simulink model "TALLER5"  (R2023b)
settings: Solver=VariableStepAuto  StartTime=0.0  StopTime=0.25  RelTol=1e-3
undefined symbols (not defined in the file): Cap, den, Kd3, Ki3, Kp2, Kp3, L, num, R
libraries: simulink x9, slpidlib x1
settings Model: Creator=Gabbi C  LastModifiedBy=Gabbi C

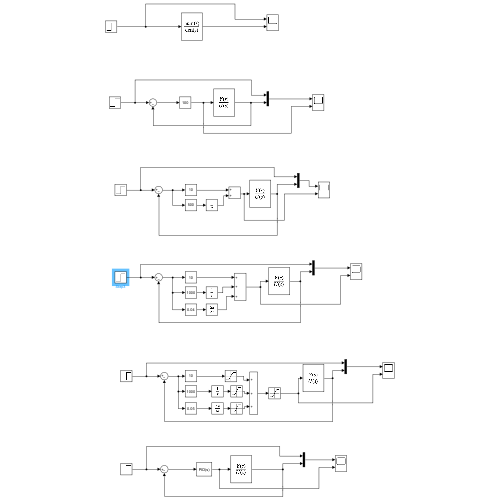
[thumbnail: Simulink's stored preview of the top-level diagram]
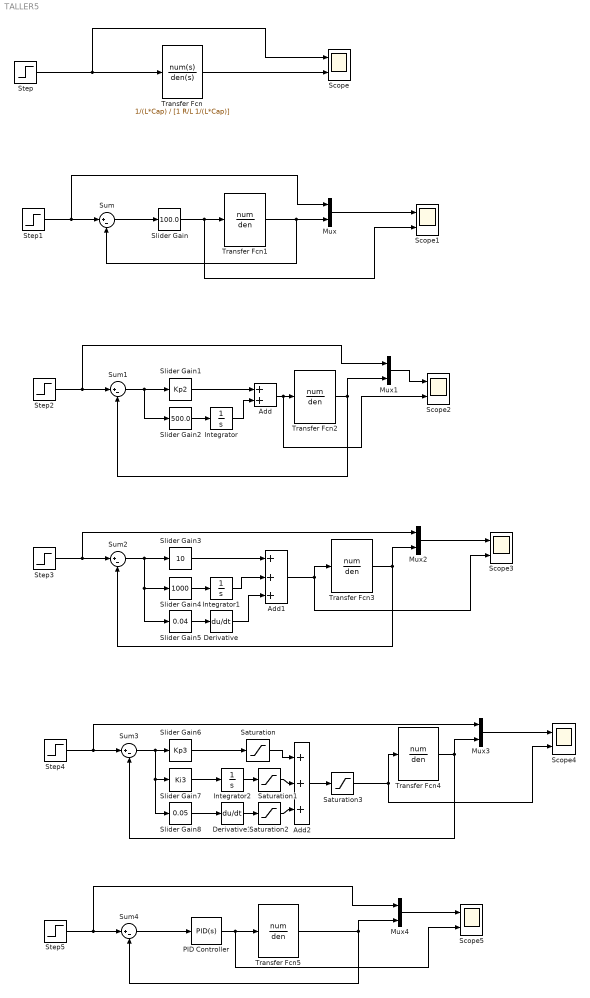
== system TALLER5 ==
  Add : Sum
  Add1 : Sum  Inputs=+++
  Add2 : Sum  Inputs=+++
  Derivative : Derivative
  Derivative1 : Derivative
  Integrator : Integrator
  Integrator1 : Integrator
  Integrator2 : Integrator
  Mux{,1..4} (5 alike) : Mux  Inputs=2
  PID Controller : slpidlib/PID Controller  Controller=PID  Form=Parallel  TimeDomain=Continuous-time  UseExternalTs=off  SampleTime=-1  IntegratorMethod=Forward Euler  FilterMethod=Forward Euler  ControllerParametersSource=internal  P=Kp3  I=Ki3  UseKiTs=off  D=Kd3  N=1000000  UseFilter=on  TunerSelectOption=Transfer Function Based (PID Tuner App)  InitialConditionSource=internal  InitialConditionForIntegrator=0  InitialConditionForFilter=0  DifferentiatorICPrevScaledInput=0  ExternalReset=none  TrackingMode=off  Kt=1  LimitOutput=off  SatLimitsSource=internal  UpperSaturationLimit=inf  LowerSaturationLimit=-inf  LinearizeAsGain=on  AntiWindupMode=none  Kb=1  LimitIntegrator=off  UpperIntegratorSaturationLimit=inf  LowerIntegratorSaturationLimit=-inf  POutMin=[]  POutMax=[]  IOutMin=[]  IOutMax=[]  DOutMin=[]  DOutMax=[]  NOutMin=[]  NOutMax=[]  SumOutMin=[]  SumOutMax=[]  SaturationOutMin=[]  SaturationOutMax=[]  PParamMin=[]  PParamMax=[]  IParamMin=[]  IParamMax=[]  DParamMin=[]  DParamMax=[]  NParamMin=[]  NParamMax=[]  KbParamMin=[]  KbParamMax=[]  KtParamMin=[]  KtParamMax=[]  KbOutMin=[]  KbOutMax=[]  KtOutMin=[]  KtOutMax=[]  IntegratorOutMin=[]  IntegratorOutMax=[]  FilterOutMin=[]  FilterOutMax=[]  SumI1OutMin=[]  SumI1OutMax=[]  SumI2OutMin=[]  SumI2OutMax=[]  SumI3OutMin=[]  SumI3OutMax=[]  SumI4OutMin=[]  SumI4OutMax=[]  SumDOutMin=[]  SumDOutMax=[]  DifferentiatorOutMin=[]  DifferentiatorOutMax=[]  FilterDiffOutCoefMin=[]  FilterDiffOutCoefMax=[]  ReciprocalOutMin=[]  ReciprocalOutMax=[]  SumDenOutMin=[]  SumDenOutMax=[]  SumNumOutMin=[]  SumNumOutMax=[]  DivideOutMin=[]  DivideOutMax=[]  UdiffTsProdOutMin=[]  UdiffTsProdOutMax=[]  NTsProdOutMin=[]  NTsProdOutMax=[]  UintegralTsProdOutMin=[]  UintegralTsProdOutMax=[]  UngainTsProdOutMin=[]  UngainTsProdOutMax=[]  ClampingZeroOutDataTypeStr=Inherit: Inherit via back propagation  ClampingZeroOutMin=[]  ClampingZeroOutMax=[]  FilterDenConstantOutDataTypeStr=Inherit: Inherit via back propagation  FilterDenConstantOutMin=[]  FilterDenConstantOutMax=[]  PCopyOutDataTypeStr=Inherit: Inherit via back propagation  PCopyOutMin=[]  PCopyOutMax=[]  NCopyOutDataTypeStr=Inherit: Inherit via back propagation  NCopyOutMin=[]  NCopyOutMax=[]  IntegratorContinuousStateAttributes=''  IntegratorStateMustResolveToSignalObject=off  IntegratorRTWStateStorageClass=Auto  FilterContinuousStateAttributes=''  FilterStateMustResolveToSignalObject=off  FilterRTWStateStorageClass=Auto  ParallelPVariant=InternalParameters  IdealPVariant=Disabled  IVariant=InternalParameters  DVariant=InternalParameters  IntegratorVariant=Continuous  SatVariant=Disabled  AWVariant=Passthrough  PCopyVariant=Disabled  TRVariant=Disabled  FdbkBlocksVariant=Forward  IdealPFdbkVariant=Disabled  SatFdbkVariant=Disabled  DerivativeFilterVariant=ContFilter  NVariant=InternalParameters  NCopyVariant=Disabled  FilterICVariant=InternalICsFilter  IntegratorICVariant=InternalICs  ExternalResetVariant=Disabled  TRSumVariant=Passthrough  SumFdbkVariant=Disabled  SumVariant=Sum_PID  TsampFilterVariant=InternalTs  TsampNgainVariant=Passthrough  TsampIntegralVariant=Disabled_SignalSpec  ExternalSaturationOutDataTypeStr=Inherit: Same as second input
  Saturation{,1..3} (4 alike) : Saturate  UpperLimit=15  LowerLimit=-15  ZeroCross=off
  Scope{,1..5} (6 alike) : Scope  NumInputPorts=2
  Slider Gain : simulink/Math Operations/Slider Gain  gain=100.0  low=0  high=100
  Slider Gain1 : simulink/Math Operations/Slider Gain  gain=Kp2  low=0  high=100
  Slider Gain2 : simulink/Math Operations/Slider Gain  gain=500.0  low=100  high=500
  Slider Gain3 : simulink/Math Operations/Slider Gain  gain=10  low=0  high=100
  Slider Gain4 : simulink/Math Operations/Slider Gain  gain=1000  low=0  high=2000
  Slider Gain5 : simulink/Math Operations/Slider Gain  gain=0.04  low=0.01  high=0.05
  Slider Gain6 : simulink/Math Operations/Slider Gain  gain=Kp3  low=0  high=100
  Slider Gain7 : simulink/Math Operations/Slider Gain  gain=Ki3  low=0  high=2000
  Slider Gain8 : simulink/Math Operations/Slider Gain  gain=0.05  low=0  high=50
  Step{,1..5} (6 alike) : Step  Time=0.01  After=5  SampleTime=0
  Sum{,1..4} (5 alike) : Sum  Inputs=|+-
  Transfer Fcn : TransferFcn  Numerator=1/(L*Cap)  Denominator=[1 R/L 1/(L*Cap)]
  Transfer Fcn{1..5} (5 alike) : TransferFcn  Numerator=num  Denominator=den
  wires:
  Step/1 -> Scope/1, Transfer Fcn/1
  Transfer Fcn/1 -> Scope/2
  Transfer Fcn1/1 -> Mux/2, Sum/2
  Step1/1 -> Mux/1, Sum/1
  Sum/1 -> Slider Gain/1
  Mux/1 -> Scope1/1
  Slider Gain/1 -> Scope1/2, Transfer Fcn1/1
  Sum1/1 -> Slider Gain2/1, Slider Gain1/1
  Transfer Fcn2/1 -> Mux1/2, Sum1/2
  Step2/1 -> Mux1/1, Sum1/1
  Mux1/1 -> Scope2/1
  Slider Gain2/1 -> Integrator/1
  Add/1 -> Scope2/2, Transfer Fcn2/1
  Slider Gain1/1 -> Add/1
  Integrator/1 -> Add/2
  Slider Gain4/1 -> Integrator1/1
  Add1/1 -> Scope3/2, Transfer Fcn3/1
  Mux2/1 -> Scope3/1
  Step3/1 -> Mux2/1, Sum2/1
  Sum2/1 -> Slider Gain5/1, Slider Gain4/1, Slider Gain3/1
  Slider Gain3/1 -> Add1/1
  Transfer Fcn3/1 -> Sum2/2, Mux2/2
  Integrator1/1 -> Add1/2
  Slider Gain5/1 -> Derivative/1
  Derivative/1 -> Add1/3
  Slider Gain8/1 -> Derivative1/1
  Add2/1 -> Saturation3/1
  Mux3/1 -> Scope4/1
  Sum3/1 -> Slider Gain8/1, Slider Gain7/1, Slider Gain6/1
  Transfer Fcn4/1 -> Sum3/2, Mux3/2
  Step4/1 -> Mux3/1, Sum3/1
  Slider Gain7/1 -> Integrator2/1
  Saturation/1 -> Add2/1
  Slider Gain6/1 -> Saturation/1
  Integrator2/1 -> Saturation1/1
  Saturation1/1 -> Add2/2
  Derivative1/1 -> Saturation2/1
  Saturation2/1 -> Add2/3
  Saturation3/1 -> Scope4/2, Transfer Fcn4/1
  PID Controller/1 -> Transfer Fcn5/1, Scope5/2
  Mux4/1 -> Scope5/1
  Step5/1 -> Mux4/1, Sum4/1
  Sum4/1 -> PID Controller/1
  Transfer Fcn5/1 -> Sum4/2, Mux4/2
